simulink model "RigidAxle_TC2024_ToBeTested"  (R2023b)
settings: Solver=VariableStepAuto  StartTime=0.0  StopTime=10.0  RelTol=1e-3
libraries: simulink x1
settings Model: Creator=joser  LastModifiedBy=joser

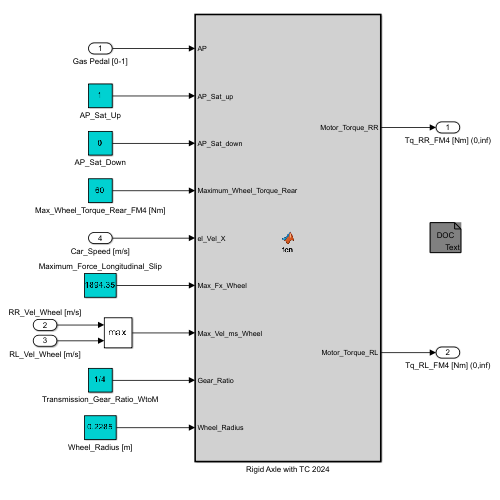
[thumbnail: Simulink's stored preview of the top-level diagram]
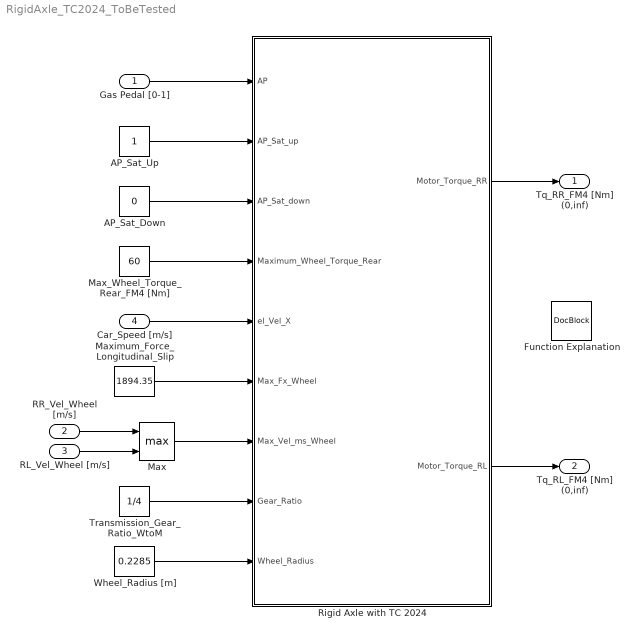
== system RigidAxle_TC2024_ToBeTested ==
  Gas Pedal [0-1] : Inport
  RR_Vel_Wheel [m/s] : Inport  Port=2
  RL_Vel_Wheel [m/s] : Inport  Port=3
  Car_Speed [m/s] : Inport  Port=4
  AP_Sat_Down : Constant  Value=0
  AP_Sat_Up : Constant
  Function Explanation : simulink/Model-Wide Utilities/DocBlock  DocumentType=Text
      content=|
      | Comparing the speed of the Ellipse and the speed of the Wheels, we can
      | determine the % of deviation between both (which is the slip). With
      | calculations from the Tyres & Performance Department, we know that the
      | maximum optimal slip in a STRAIGHT line is 15%. Therefore (using the Magic
      | Formula), we can determine the maximum X-Force permissible by the Wheels
      | with that % of slip (which is the constant Max_Fx_Tyre, input
      | of Rigid Axle).
      |
      | With that and the radius of the Wheels, we can calculate the maximum
      | Torque for it to stop slipping.
  Max : MinMax  Function=max  Inputs=2
  Max_Wheel_Torque_Rear_FM4 [Nm] : Constant  Value=60
  Maximum_Force_Longitudinal_Slip : Constant  Value=1894.35
  "Rigid Axle with TC 2024 " : MATLAB Function  TreatAsAtomicUnit=on
  Transmission_Gear_Ratio_WtoM : Constant  Value=1/4
  Wheel_Radius [m] : Constant  Value=0.2285
  Tq_RR_FM4 [Nm] (0,inf) : Outport  VectorParamsAs1DForOutWhenUnconnected=off
  Tq_RL_FM4 [Nm] (0,inf) : Outport  Port=2  VectorParamsAs1DForOutWhenUnconnected=off
  wires:
  Max/1 -> "Rigid Axle with TC 2024 "/7(Max_Vel_ms_Wheel)
  Wheel_Radius [m]/1 -> "Rigid Axle with TC 2024 "/9(Wheel_Radius)
  RL_Vel_Wheel [m/s]/1 -> Max/2
  AP_Sat_Up/1 -> "Rigid Axle with TC 2024 "/2(AP_Sat_up)
  Maximum_Force_Longitudinal_Slip/1 -> "Rigid Axle with TC 2024 "/6(Max_Fx_Wheel)
  "Rigid Axle with TC 2024 "/2(Motor_Torque_RL) -> Tq_RL_FM4 [Nm] (0,inf)/1
  "Rigid Axle with TC 2024 "/1(Motor_Torque_RR) -> Tq_RR_FM4 [Nm] (0,inf)/1
  RR_Vel_Wheel [m/s]/1 -> Max/1
  AP_Sat_Down/1 -> "Rigid Axle with TC 2024 "/3(AP_Sat_down)
  Transmission_Gear_Ratio_WtoM/1 -> "Rigid Axle with TC 2024 "/8(Gear_Ratio)
  Max_Wheel_Torque_Rear_FM4 [Nm]/1 -> "Rigid Axle with TC 2024 "/4(Maximum_Wheel_Torque_Rear)
  Gas Pedal [0-1]/1 -> "Rigid Axle with TC 2024 "/1(AP)
  Car_Speed [m/s]/1 -> "Rigid Axle with TC 2024 "/5(el_Vel_X)

== matlab function RigidAxle_TC2024_ToBeTested/Rigid Axle with TC 2024  ==
  data: AP input; Motor_Torque_RR output; AP_Sat_up input; AP_Sat_down input; Maximum_Wheel_Torque_Rear input; Motor_Torque_RL output; el_Vel_X input; Max_Fx_Wheel input; Max_Vel_ms_Wheel input; Gear_Ratio input; Wheel_Radius input
function [Motor_Torque_RR, Motor_Torque_RL] = fcn(AP, AP_Sat_up, AP_Sat_down, Maximum_Wheel_Torque_Rear, el_Vel_X, Max_Fx_Wheel, Max_Vel_ms_Wheel, Gear_Ratio, Wheel_Radius)

Slip = Max_Vel_ms_Wheel / el_Vel_X; % Percentage of slip
    %% Accelerator pedal with saturations

    if AP <= AP_Sat_down

        Throttle = 0; % If the real position of the pedal is lower than the minimum saturation --> lifted throttle.
        Pedal_pressed = 0;

    elseif AP >= AP_Sat_up

        Throttle = 1;  % If the real position of the pedal is higher than the maximum saturation --> full throttle.
        Pedal_pressed = 1;
    
    else
        Throttle = (AP - AP_Sat_down)/(AP_Sat_up - AP_Sat_down); % Compute the percentage of pedal pressed (if it is not 1 or 0) regarding the maximun and minimum saturation
        Pedal_pressed = 1;
    
    end

    %% Motor Torque

    if Slip < 1.15 % 15% of slip, greater than that number it is not optimal.

        Motor_Torque_RR = Maximum_Wheel_Torque_Rear * Gear_Ratio * Throttle; % Rear Right (RR) motor torque output.
        Motor_Torque_RL = Maximum_Wheel_Torque_Rear * Gear_Ratio * Throttle; % Rear Left (RL) motor torque output.
        % Percentage of Pedal = final percentage of Torque (referenced to Maximum_Torque_Rear).

    else 
        Motor_Torque_RR = Max_Fx_Wheel * Wheel_Radius * Gear_Ratio * Pedal_pressed; % Motor Torque RR output if tyre slips more than 15%.
        Motor_Torque_RL = Max_Fx_Wheel * Wheel_Radius * Gear_Ratio * Pedal_pressed; % Motor Torque RL output if tyre slips more than 15%.

        % EXPLANATION:
        % Max_Fx_Wheel * Wheel_Radius * Gear_ratio = 
        % = Max_Torque_Wheel * Gear_Ratio =
        % = Torque_Motor
        % Max_Fx_Tyre got it with Magic Formula MATLAB (Tyres & Performance guys) 
        % More information at the Doc outside the function.
        
    end
end
